simulink model "lab3"  (Simulink 9.2)
settings: Solver=VariableStepAuto  StartTime=0.0  StopTime=80.0  RelTol=1e-3
settings Model: Creator=Елена  LastModifiedBy=Елена
settings DataIOCC: LimitDataPoints=off  SaveFormat=Dataset  SignalLoggingSaveFormat=Dataset
settings OptimizationCC: LifeSpan=auto
settings DebuggingCC: UnderspecifiedInitializationDetection=Simplified  MergeDetectMultiDrivingBlocksExec=error  FcnCallInpInsideContextMsg=error  StateNameClashWarn=none  SFUnexpectedBacktrackingDiag=error  SFNoUnconditionalDefaultTransitionDiag=error  SFExecutionAtInitializationDiag=warning
settings HardwareCC: ProdBitPerPointer=64  ProdBitPerSizeT=64  ProdBitPerPtrDiffT=64  ProdLargestAtomicFloat=Float  ProdIntDivRoundTo=Zero  ProdEndianess=LittleEndian  ProdWordSize=64  ProdHWDeviceType=Intel->x86-64 (Windows64)
settings ModelReferenceCC: PropagateSignalLabelsOutOfModel=on
settings SFSimCC: SimUseLocalCustomCode=on
settings RTWCC: RTWUseLocalCustomCode=on
settings CodeAppCC: StateflowObjectComments=off
settings GRTTargetCC: TargetLangStandard=C99 (ISO)  GeneratePreprocessorConditionals=Use local settings  CombineOutputUpdateFcns=on  GRTInterface=off
settings ConfigComp: CovMetricSettings=dwe  CovHtmlReporting=off  CovSaveCumulativeToWorkspaceVar=off  CovSaveSingleToWorkspaceVar=off  CovExternalEMLEnable=on

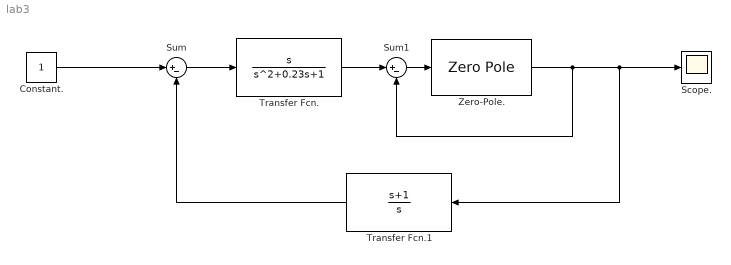
== system lab3 ==
  Constant. : Constant
  Scope. : Scope
  Sum : Sum  Inputs=|+-
  Sum1 : Sum  Inputs=|+-
  Transfer Fcn. : TransferFcn  Numerator=[1 0]  Denominator=[1 0.23 1]
  Transfer Fcn.1 : TransferFcn  Numerator=[1 1]  Denominator=[ 1 0]
  Zero-Pole. : ZeroPole  Zeros=[0]  Poles=[-0.09 -1]
  wires:
  Constant./1 -> Sum/1
  Sum/1 -> Transfer Fcn./1
  Zero-Pole./1 -> Scope./1, Transfer Fcn.1/1, Sum1/2
  Transfer Fcn./1 -> Sum1/1
  Sum1/1 -> Zero-Pole./1
  Transfer Fcn.1/1 -> Sum/2
